simulink model "scara_controller_speed_control"  (R2013a)
settings: Solver=ode1  SolverMode=SingleTasking  StartTime=0.0  StopTime=inf  RelTol=1e-3
PreLoadFcn:
  | waijung.modelPreload; % Required for working with Waijung Blockset. Do not remove.
undefined symbols (not defined in the file or in its folder): ARM, disable_customio, enable_customio, fdesignblkfcn, gcbh, in1, in2, Link, LQFP100, MDK, out1, out2, out3, out4, out5, out6, output_customio, ST, STM32F407VG, STM32F4DISCOVERY
libraries: simulink x6, stm32f4_io_lib x3, USBVCP_STM32F4 x2, waijung_customcode x1, stm32f4_adc_lib x1, stm32f4_device_config_lib x1
CloseFcn:
  | waijung.modelClose; % Required for working with Waijung Blockset. Do not remove.
settings Model: Creator=Sr Antonio  LastModifiedBy=sp
settings DataIOCC: SignalLoggingSaveFormat=ModelDataLogs
settings OptimizationCC: ExpressionDepthLimit=2147483647  OptimizeModelRefInitCode=on  LifeSpan=1
settings DebuggingCC: MultiTaskDSMMsg=warning  FcnCallInpInsideContextMsg=EnableAllAsWarning
settings HardwareCC: ProdEndianess=LittleEndian  ProdHWDeviceType=ARM Compatible->Cortex - M4  TargetEndianess=LittleEndian  TargetHWDeviceType=ARM Compatible->Cortex - M4
settings RTWCC: SystemTargetFile=stm32f4.tlc  GenerateMakefile=off  TemplateMakefile=ert_default_tmf  Description=STM32F4 Target  ProcessScript=stm32f4_make_rtw_hook  RTWUseSimCustomCode=on
settings CodeAppCC: IgnoreCustomStorageClasses=off  CustomSymbolStrType=$N$R$M  InternalIdentifier=Classic
settings STFCustomTargetCC: ModelReferenceCompliant=off  CombineOutputUpdateFcns=on  ERTCustomFileBanners=on  SupportNonInlinedSFcns=off  MATLABClassNameForMDSCustomization=Simulink.SoftwareTarget.ERTCustomization  SystemTargetFile=stm32f4.tlc
settings ERTTargetCC: GenerateSampleERTMain=off  ModelReferenceCompliant=off  ParMdlRefBuildCompliant=off  CompOptLevelCompliant=off  ConcurrentExecutionCompliant=off  ERTFirstTimeCompliant=off  SupportContinuousTime=on  ModelStepFunctionPrototypeControlCompliant=off  CPPClassGenCompliant=off  ExtModeMexFile=noextcomm  ERTSrcFileBannerTemplate=stm32f4_code_template.cgt  ERTHdrFileBannerTemplate=stm32f4_code_template.cgt  ERTDataSrcFileTemplate=stm32f4_code_template.cgt  ERTDataHdrFileTemplate=stm32f4_code_template.cgt  ERTCustomFileTemplate=stm32f4_file_process.tlc

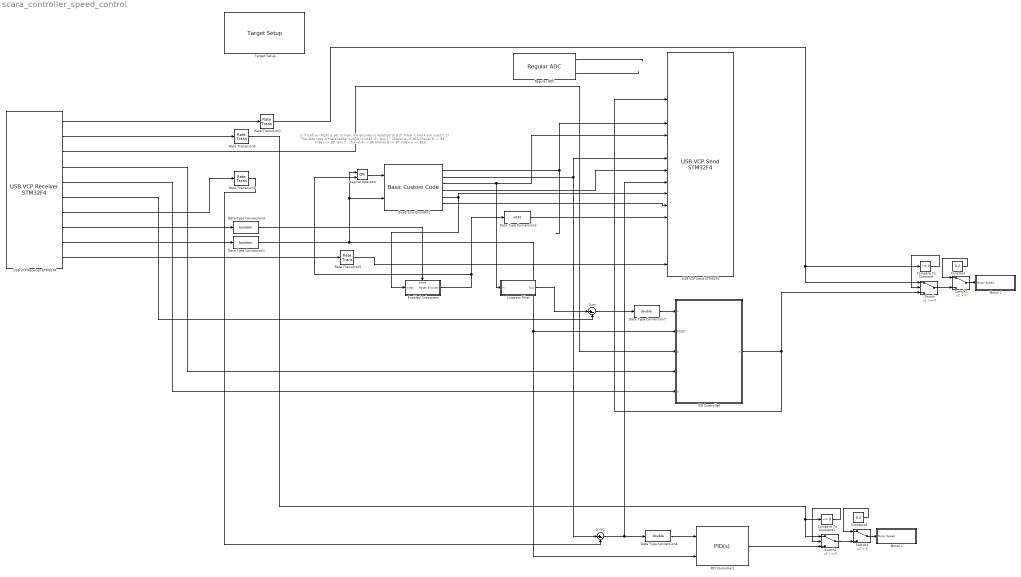
== system scara_controller_speed_control ==
  note: 1) if rLeft or rRight is set to high, the encoder is resetted to 0
      | 2) Timer 2 and 4 are used!!!
      | 2) The data type of the encoder output is int32.
      | 3) "enc 1": 	Chanel A --> A15
      | 		       Chanel B --> B3
      | 			Index --> D0
      |   "enc 2": 	Chanel A --> B6
      | 		       Chanel B --> B7
      | 			Index-> --> B12
  Compare To Constant : simulink/Logic and Bit Operations/Compare To Constant  relop=~=  const=0  OutDataTypeStr=boolean
  Compare To Constant1 : simulink/Logic and Bit Operations/Compare To Constant  relop=~=  const=0  OutDataTypeStr=boolean
  Constant : Constant  Value=0.2
  Constant2 : Constant  Value=0.2
  Data Type Conversion1 : DataTypeConversion  OutDataTypeStr=boolean
  Data Type Conversion2 : DataTypeConversion  OutDataTypeStr=int32
  Data Type Conversion3 : DataTypeConversion  OutDataTypeStr=boolean
  Data Type Conversion4 : DataTypeConversion  OutDataTypeStr=double
  Data Type Conversion7 : DataTypeConversion  OutDataTypeStr=double
  Enabled Subsystem : Subsystem  TreatAsAtomicUnit=on
  Logical Operator : Logic  Operator=OR  AllPortsSameDT=off  OutDataTypeStr=boolean
  Lowpass Filter : Subsystem  DialogController=fdesignblkfcn  InitFcn=fdesignblkfcn(gcbh, {'InitFcn'});  mask(Lowpass Filter){}
      mask help: Design a lowpass filter
      settings: CopyFcn=fdesignblkfcn(gcbh, {'CopyFcn'});
      mask Help: helpview(mapfilelocation('dsp'), 'dsplowpassfilter');
      mask Display: disp('Lowpass')
  Motor 1 : Subsystem
  Motor 2 : Subsystem
  PID Controller : Subsystem  DialogController=pidpack.PIDConfig.pidDDGCreate  mask(PID 1dof){Controller=PID, TimeDomain=Continuous-time, SampleTime=1, IntegratorMethod=Forward Euler, FilterMethod=Forward Euler, Form=Parallel, P=0.0005, I=0.0005, D=0, N=20, InitialConditionSource=internal, InitialConditionForIntegrator=0, InitialConditionForFilter=0, ExternalReset=rising, IgnoreLimit=off, ZeroCross=on, LimitOutput=on, UpperSaturationLimit=1, LowerSaturationLimit=-1, LinearizeAsGain=on, AntiWindupMode=clamping, Kb=1, TrackingMode=off, Kt=1, RndMeth=Floor, SaturateOnIntegerOverflow=off, LockScale=off, PParamMin=[], PParamMax=[], PParamDataTypeStr=Inherit: Inherit via internal rule, IParamMin=[], IParamMax=[], IParamDataTypeStr=Inherit: Inherit via internal rule, DParamMin=[], DParamMax=[], DParamDataTypeStr=Inherit: Inherit via internal rule, NParamMin=[], NParamMax=[], NParamDataTypeStr=Inherit: Inherit via internal rule, KbParamMin=[], KbParamMax=[], KbParamDataTypeStr=Inherit: Inherit via internal rule, KtParamMin=[], KtParamMax=[], KtParamDataTypeStr=Inherit: Inherit via internal rule, POutMin=[], POutMax=[], POutDataTypeStr=Inherit: Inherit via internal rule, IOutMin=[], IOutMax=[], IOutDataTypeStr=Inherit: Inherit via internal rule, DOutMin=[], DOutMax=[], DOutDataTypeStr=Inherit: Inherit via internal rule, NOutMin=[], NOutMax=[], NOutDataTypeStr=Inherit: Inherit via internal rule, KbOutMin=[], KbOutMax=[], KbOutDataTypeStr=Inherit: Inherit via internal rule, KtOutMin=[], KtOutMax=[], KtOutDataTypeStr=Inherit: Inherit via internal rule, IntegratorOutMin=[], IntegratorOutMax=[], IntegratorOutDataTypeStr=Inherit: Inherit via internal rule, FilterOutMin=[], FilterOutMax=[], FilterOutDataTypeStr=Inherit: Inherit via internal rule, SumOutMin=[], SumOutMax=[], SumOutDataTypeStr=Inherit: Inherit via internal rule, SumI1OutMin=[], SumI1OutMax=[], SumI1OutDataTypeStr=Inherit: Inherit via internal rule, SumI2OutMin=[], SumI2OutMax=[], SumI2OutDataTypeStr=Inherit: Inherit via internal rule, SumI3OutMin=[], SumI3OutMax=[], SumI3OutDataTypeStr=Inherit: Inherit via internal rule, SumDOutMin=[], SumDOutMax=[], SumDOutDataTypeStr=Inherit: Inherit via internal rule, SumAccumDataTypeStr=Inherit: Inherit via internal rule, SumI1AccumDataTypeStr=Inherit: Inherit via internal rule, SumI2AccumDataTypeStr=Inherit: Inherit via internal rule, SumI3AccumDataTypeStr=Inherit: Inherit via internal rule, SumDAccumDataTypeStr=Inherit: Inherit via internal rule, SaturationOutMin=[], SaturationOutMax=[], SaturationOutDataTypeStr=Inherit: Same as input, IntegratorContinuousStateAttributes='', IntegratorStateIdentifier=, IntegratorStateMustResolveToSignalObject=off, IntegratorRTWStateStorageClass=Auto, IntegratorRTWStateStorageTypeQualifier=, FilterContinuousStateAttributes='', FilterStateIdentifier=, FilterStateMustResolveToSignalObject=off, FilterRTWStateStorageClass=Auto, FilterRTWStateStorageTypeQualifier=}
      mask prompts: Controller "Simulink:masks:Controller_MP"; TimeDomain "Simulink:masks:TimeDomain_MP"; SampleTime "Simulink:masks:SampleTime1ForInherited_MP"; IntegratorMethod "Simulink:masks:IntegratorMethod_MP"; FilterMethod "Simulink:masks:FilterMethod_MP"; Form "Simulink:masks:Form_MP"; P "Simulink:masks:ProportionalP_MP"; I "Simulink:masks:IntegralI_MP"; D "Simulink:masks:DerivativeD_MP"; N "Simulink:masks:FilterCoefficientN_MP"; InitialConditionSource "Simulink:masks:Source_MP"; InitialConditionForIntegrator "Simulink:masks:Integrator_MP"; InitialConditionForFilter "Simulink:masks:Filter_MP"; ExternalReset "Simulink:masks:ExternalReset_MP"; IgnoreLimit "Simulink:masks:IgnoreResetWhenLinearizing_MP"; ZeroCross "Simulink:masks:EnableZerocrossingDetection_MP"; LimitOutput "Simulink:masks:LimitOutput_MP"; UpperSaturationLimit "Simulink:masks:UpperSaturationLimit_MP"; LowerSaturationLimit "Simulink:masks:LowerSaturationLimit_MP"; LinearizeAsGain "Simulink:masks:IgnoreSaturationWhenLinearizing_MP"; AntiWindupMode "Simulink:masks:AntiwindupMethod_MP"; Kb "Simulink:masks:BackcalculationCoefficientKb_MP"; TrackingMode "Simulink:masks:EnableTrackingMode_MP"; Kt "Simulink:masks:TrackingCoefficientKt_MP"; RndMeth "Simulink:masks:IntegerRoundingMode_MP"; SaturateOnIntegerOverflow "Simulink:masks:SaturateOnIntegerOverflow_MP"; LockScale "Simulink:masks:LockDataTypeAgainstFxpTools_MP"; PParamMin "Simulink:masks:PParameterMinimum_MP"; PParamMax "Simulink:masks:PParameterMaximum_MP"; PParamDataTypeStr "Simulink:masks:PParameter_MP"; IParamMin "Simulink:masks:IParameterMinimum_MP"; IParamMax "Simulink:masks:IParameterMaximum_MP"; IParamDataTypeStr "Simulink:masks:IParameter_MP"; DParamMin "Simulink:masks:DParameterMinimum_MP"; DParamMax "Simulink:masks:DParameterMaximum_MP"; DParamDataTypeStr "Simulink:masks:DParameter_MP"; NParamMin "Simulink:masks:NParameterMinimum_MP"; NParamMax "Simulink:masks:NParameterMaximum_MP"; NParamDataTypeStr "Simulink:masks:NParameter_MP"; KbParamMin "Simulink:masks:KbParameterMinimum_MP"; KbParamMax "Simulink:masks:KbParameterMaximum_MP"; KbParamDataTypeStr "Simulink:masks:KbParameter_MP"; KtParamMin "Simulink:masks:KtParameterMinimum_MP"; KtParamMax "Simulink:masks:KtParameterMaximum_MP"; KtParamDataTypeStr "Simulink:masks:KtParameter_MP"; POutMin "Simulink:masks:PProductOutputMinimum_MP"; POutMax "Simulink:masks:PProductOutputMaximum_MP"; POutDataTypeStr "Simulink:masks:PProductOutput_MP"; IOutMin "Simulink:masks:IProductOutputMinimum_MP"; IOutMax "Simulink:masks:IProductOutputMaximum_MP"; IOutDataTypeStr "Simulink:masks:IProductOutput_MP"; DOutMin "Simulink:masks:DProductOutputMinimum_MP"; DOutMax "Simulink:masks:DProductOutputMaximum_MP"; DOutDataTypeStr "Simulink:masks:DProductOutput_MP"; NOutMin "Simulink:masks:NProductOutputMinimum_MP"; NOutMax "Simulink:masks:NProductOutputMaximum_MP"; NOutDataTypeStr "Simulink:masks:NProductOutput_MP"; KbOutMin "Simulink:masks:KbProductOutputMinimum_MP"; KbOutMax "Simulink:masks:KbProductOutputMaximum_MP"; KbOutDataTypeStr "Simulink:masks:KbProductOutput_MP"; KtOutMin "Simulink:masks:KtProductOutputMinimum_MP"; KtOutMax "Simulink:masks:KtProductOutputMaximum_MP"; KtOutDataTypeStr "Simulink:masks:KtProductOutput_MP"; IntegratorOutMin "Simulink:masks:IntegratorOutputMinimum_MP"; IntegratorOutMax "Simulink:masks:IntegratorOutputMaximum_MP"; IntegratorOutDataTypeStr "Simulink:masks:IntegratorOutput_MP"; FilterOutMin "Simulink:masks:FilterOutputMinimum_MP"; FilterOutMax "Simulink:masks:FilterOutputMaximum_MP"; FilterOutDataTypeStr "Simulink:masks:FilterOutput_MP"; SumOutMin "Simulink:masks:SumOutputMinimum_MP"; SumOutMax "Simulink:masks:SumOutputMaximum_MP"; SumOutDataTypeStr "Simulink:masks:SumOutput_MP"; SumI1OutMin "Simulink:masks:SumI1OutputMinimum_MP"; SumI1OutMax "Simulink:masks:SumI1OutputMaximum_MP"; SumI1OutDataTypeStr "Simulink:masks:SumI1Output_MP"; SumI2OutMin "Simulink:masks:SumI2OutputMinimum_MP"; SumI2OutMax "Simulink:masks:SumI2OutputMaximum_MP"; SumI2OutDataTypeStr "Simulink:masks:SumI2Output_MP"; SumI3OutMin "Simulink:masks:SumI3OutputMinimum_MP"; SumI3OutMax "Simulink:masks:SumI3OutputMaximum_MP"; SumI3OutDataTypeStr "Simulink:masks:SumI3Output_MP"; SumDOutMin "Simulink:masks:SumDOutputMinimum_MP"; SumDOutMax "Simulink:masks:SumDOutputMaximum_MP"; SumDOutDataTypeStr "Simulink:masks:SumDOutput_MP"; SumAccumDataTypeStr "Simulink:masks:AccumulatorOfSum_MP"; SumI1AccumDataTypeStr "Simulink:masks:AccumulatorOfSumI1_MP"; SumI2AccumDataTypeStr "Simulink:masks:AccumulatorOfSumI2_MP"; SumI3AccumDataTypeStr "Simulink:masks:AccumulatorOfSumI3_MP"; SumDAccumDataTypeStr "Simulink:masks:AccumulatorOfSumD_MP"; SaturationOutMin "Simulink:masks:SaturationOutputMinimum_MP"; SaturationOutMax "Simulink:masks:SaturationOutputMaximum_MP"; SaturationOutDataTypeStr "Simulink:masks:SaturationOutput_MP"; IntegratorContinuousStateAttributes "Simulink:masks:StateNameegposition_MP"; IntegratorStateIdentifier "Simulink:masks:StateName_MP"; IntegratorStateMustResolveToSignalObject "Simulink:masks:StateNameMustResolveToSimulinkSignalObject_MP"; IntegratorRTWStateStorageClass "Simulink:masks:CodeGenerationStorageClass_MP"; IntegratorRTWStateStorageTypeQualifier "Simulink:masks:CodeGenerationStorageTypeQualifier_MP"; FilterContinuousStateAttributes "Simulink:masks:StateNameegposition_MP"; FilterStateIdentifier "Simulink:masks:StateName_MP"; FilterStateMustResolveToSignalObject "Simulink:masks:StateNameMustResolveToSimulinkSignalObject_MP"; FilterRTWStateStorageClass "Simulink:masks:CodeGenerationStorageClass_MP"; FilterRTWStateStorageTypeQualifier "Simulink:masks:CodeGenerationStorageTypeQualifier_MP"
      mask help: Simulink:masks:PID1dof_MD
      mask init:
      | pidpack.PIDConfig.configPID(gcbh);
      settings: DeleteFcn=pidpack.PIDConfig.closeTuner(gcbh)  ModelCloseFcn=pidpack.PIDConfig.closeTuner(gcbh)  NameChangeFcn=pidpack.PIDConfig.updateTunerName(gcbh)
      mask TypeOptions Controller: Simulink:masks:PID | Simulink:masks:PI | Simulink:masks:PD | Simulink:masks:P | Simulink:masks:I
      mask TypeOptions TimeDomain: Simulink:masks:ContinuousTime | Simulink:masks:DiscreteTime
      mask TypeOptions IntegratorMethod: Simulink:masks:ForwardEuler | Simulink:masks:BackwardEuler | Simulink:masks:Trapezoidal
      mask TypeOptions FilterMethod: Simulink:masks:ForwardEuler | Simulink:masks:BackwardEuler | Simulink:masks:Trapezoidal
      mask TypeOptions Form: Simulink:masks:Ideal | Simulink:masks:Parallel
      mask TypeOptions InitialConditionSource: Simulink:masks:internal | Simulink:masks:external
      mask TypeOptions ExternalReset: Simulink:masks:none | Simulink:masks:rising | Simulink:masks:falling | Simulink:masks:either | Simulink:masks:level
      mask TypeOptions AntiWindupMode: Simulink:masks:none | Simulink:masks:backCalculation | Simulink:masks:clamping
      mask TypeOptions RndMeth: Simulink:masks:Ceiling | Simulink:masks:Convergent | Simulink:masks:Floor | Simulink:masks:Nearest | Simulink:masks:Round | Simulink:masks:Simplest | Simulink:masks:Zero
      mask TypeOptions IntegratorRTWStateStorageClass: Simulink:masks:Auto | Simulink:masks:ExportedGlobal | Simulink:masks:ImportedExtern | Simulink:masks:ImportedExternPointer
      mask TypeOptions FilterRTWStateStorageClass: Simulink:masks:Auto | Simulink:masks:ExportedGlobal | Simulink:masks:ImportedExtern | Simulink:masks:ImportedExternPointer
      mask Display:
      | image(imread(fullfile(matlabroot,'toolbox','simulink','blocks','@pidpack','@PIDMasks','images','blank.png'),'png'),[0 0 1 1]);
      | disp('PID(s)')
      | port_label('input',1, '');
      | port_label('output',1, '');
      | plot([0 4 4 7]+2,[0 0 8 8]+208);
      | plot([1 4 6]+2,[3 6 3]+208);
      | plot([0 4 6 10]+182,[0 0 8 8]+148);
  PID Controller1 : simulink/Continuous/PID Controller  Controller=PID  TimeDomain=Continuous-time  SampleTime=1  IntegratorMethod=Forward Euler  FilterMethod=Forward Euler  Form=Parallel  P=0.0005  I=0.0005  D=0  N=100  InitialConditionSource=internal  InitialConditionForIntegrator=0  InitialConditionForFilter=0  ExternalReset=rising  LimitOutput=on  UpperSaturationLimit=1  LowerSaturationLimit=-1  LinearizeAsGain=on  AntiWindupMode=clamping  Kb=1  TrackingMode=off  Kt=1  PParamMin=[]  PParamMax=[]  IParamMin=[]  IParamMax=[]  DParamMin=[]  DParamMax=[]  NParamMin=[]  NParamMax=[]  KbParamMin=[]  KbParamMax=[]  KtParamMin=[]  KtParamMax=[]  POutMin=[]  POutMax=[]  IOutMin=[]  IOutMax=[]  DOutMin=[]  DOutMax=[]  NOutMin=[]  NOutMax=[]  KbOutMin=[]  KbOutMax=[]  KtOutMin=[]  KtOutMax=[]  IntegratorOutMin=[]  IntegratorOutMax=[]  FilterOutMin=[]  FilterOutMax=[]  SumOutMin=[]  SumOutMax=[]  SumI1OutMin=[]  SumI1OutMax=[]  SumI2OutMin=[]  SumI2OutMax=[]  SumI3OutMin=[]  SumI3OutMax=[]  SumDOutMin=[]  SumDOutMax=[]  SaturationOutMin=[]  SaturationOutMax=[]  IntegratorContinuousStateAttributes=''  IntegratorStateMustResolveToSignalObject=off  IntegratorRTWStateStorageClass=Auto  FilterContinuousStateAttributes=''  FilterStateMustResolveToSignalObject=off  FilterRTWStateStorageClass=Auto
  Quadratur Encoder2 : waijung_customcode/Basic Custom Code  inputporttype=boolean,boolean  cinputportlabel=resetEncoder1, resetEncoder2  cinputportlabelstr="[\"resetEncoder1\",\" resetEncoder2\"]"  inputportcount=2  inputporttypeid="[8  8]"  outputporttype=int32,int32,int32,int32,int32,int32  coutputportlabel=encoder1, encoder2, encoder1_speed, encoder2_speed, encoder1_index, encoder2_index  coutputportlabelstr="[\"encoder1\",\" encoder2\",\" encoder1_speed\",\" encoder2_speed\",\" encoder1_index\",\" encoder2_index\"]"  outputportcount=6  outputporttypeid="[6  6  6  6  6  6]"  incpath={fullfile(pwd,'customcode')}  srcpath={fullfile(pwd,'customcode')}  incfiles={''}  srcfiles={'stm32f4_io_customcode.c'}  enablefuncallstr=enable_customio();  outputfuncallstr=output_customio(in1,in2,out1,out2,out3,out4,out5,out6);  disablefuncallstr=disable_customio();  sampletime=0.001  sampletimestr=0.001  blockid=QuadraturEncoder2  enablecustomportlabel=on  incfilestrarray="[\"\"]"  inputportdiminfo="[1  1  1  8;1  1  1  8]"  outputportdiminfo="[1  1  1  6;1  1  1  6;1  1  1  6;1  1  1  6;1  1  1  6;1  1  1  6]"
  Rate Transition1 : RateTransition  Integrity=off  Deterministic=off  OutPortSampleTime=0.001
  Rate Transition3 : RateTransition  OutPortSampleTime=0.01
  Rate Transition4 : RateTransition  Integrity=off  Deterministic=off  OutPortSampleTime=0.001
  Rate Transition5 : RateTransition  OutPortSampleTime=0.01
  Regular ADC : stm32f4_adc_lib/Regular ADC  adcmodule=1  outputdatatype=Double  prescaler=2  prescalerstr=ADC_Prescaler_Div2  chsamplingtime=Auto  chsamplingtimestr=ADC_SampleTime_480Cycles  read_an0=off  read_an1=off  read_an2=off  read_an3=off  read_an4=off  read_an5=on  read_an6=off  read_an7=off  read_an8=off  read_an9=off  read_an10=off  read_an11=off  read_an12=off  read_an13=off  read_an14=off  read_an15=off  read_an16=off  read_an17=on  read_an18=off  pinstr=GPIO_Pin_5  usedpinarray="[0  0  0  0  0  1  0  0  0  0  0  0  0  0  0  0  0  1  0]"  usedportidarray=[0]  usedpinidarray=[5]  usedpinidcount=1  sampletime=0.01  blockid=RegularADC  enablecustomportlabel=on  cinputportlabel=0  coutputportlabel=Motor1Current, BoardTemp
  Sum : Sum  Inputs=|+-  AccumDataTypeStr=int32
  Sum1 : Sum  Inputs=|+-  AccumDataTypeStr=int32
  Switch : Switch
  Switch1 : Switch
  Switch2 : Switch  Criteria=u2 > Threshold
  Switch4 : Switch  Criteria=u2 > Threshold
  Target Setup : stm32f4_device_config_lib/Target Setup  Priority=100  compiler=MDK-ARM  previous_compiler=MDK-ARM  mcu=STM32F407VG (LQFP100); STM32F4DISCOVERY  mcustr=STM32F407VG  clockconfig=STM32F4DISCOVERY Default (HSEOSC-8MHz/HCLK-168MHz)  system_stm32f4xx_c_path=C:\Program Files\MATLAB\waijung14_12a\targets\stm32f4_target\stm32f4\utils\STM32F4xx_AN3988_V1.0.1\stm32f4_default\hseosc8mhz  showmemoryconfiguration=on  stacksize=0x2000  heapsize=0x2000  enableautocompiledownload=on  fullchiperase=off  programmerinterface=ST-Link  editctrlstr=on  compilercontrolstr=-c --cpu Cortex-M4.fp -g -O3 --apcs=interwork --split_sections $(INCLUDES)  assemblercontrolstr="--cpu Cortex-M4.fp -g --apcs=interwork  --xref $(INCLUDES)"  linkercontrolstr="--cpu Cortex-M4.fp --strict --scatter \"$(MODELNAME).sct\" --summary_stderr --info summarysizes --map --xref --callgraph --symbols --info sizes --info totals --info unused --info veneers  --list \".\\$(MODELNAME).map\" -o $(MODELNAME).axf"  runafterdownload=on  execprofile=None  profileruart=1  profilerbaud=115200  profilertxpin=Not used  profilerinitstr=0.001,168000000,168000,115200,0  manualsetsampletime=off  sampletime=0.001  blockid=TargetSetup  systickreloadvalue=168000  hseval=8000000  lastprofileruart=1  hclk=168000000  flashorigin=0x08000000  flashlength=0x00100000  ramorigin=0x20000000  ramlength=0x00020000  useextram=off
  USB VCP Receiver STM32F4 : USBVCP_STM32F4/USB VCP Receiver STM32F4  speed="USB 1.1   12Mbit/s"  data_size=2048 Bytes  header_data='7E 7E'  binary_data='double double double double double int32 int32 int32 int32 int32'  terminator_data='03 03'  sampletime=0.001
  USB VCP Send STM32F1 : USBVCP_STM32F4/USB VCP Send STM32F4  speed="USB 1.1   12Mbit/s"  data_size=2048 Bytes  header_data='0E 0E'  binary_data='double double double double int32 int32 int32 int32 int32 int32 int32 int32 int32 int32 int32 int32 int32 int32'  terminator_data='0A 0A'  sampletime=0.001
  wires:
  USB VCP Receiver STM32F4/1 -> Rate Transition1/1
  Quadratur Encoder2/1 -> USB VCP Send STM32F1/6
  PID Controller/1(y) -> Switch/3, USB VCP Send STM32F1/4
  Sum/1 -> Data Type Conversion7/1
  Switch/1 -> Switch2/3
  Compare To Constant/1 -> Switch/2
  Quadratur Encoder2/2 -> USB VCP Send STM32F1/9, Sum1/1
  PID Controller1/1 -> Switch1/3
  Rate Transition3/1 -> Sum1/2
  Sum1/1 -> Data Type Conversion4/1, USB VCP Send STM32F1/11
  Data Type Conversion4/1 -> PID Controller1/1
  Data Type Conversion1/1 -> Quadratur Encoder2/2, Logical Operator/1, PID Controller1/2, PID Controller/2(RESET)
  Switch1/1 -> Switch4/3
  Compare To Constant1/1 -> Switch1/2
  USB VCP Receiver STM32F4/7 -> Rate Transition3/1
  USB VCP Receiver STM32F4/2 -> Rate Transition4/1
  USB VCP Receiver STM32F4/9 -> Data Type Conversion1/1
  Quadratur Encoder2/3 -> USB VCP Send STM32F1/7, Lowpass Filter/1(In)
  Quadratur Encoder2/4 -> USB VCP Send STM32F1/10
  Rate Transition1/1 -> Switch/1, Compare To Constant/1
  Rate Transition4/1 -> Switch1/1, Compare To Constant1/1
  Data Type Conversion7/1 -> PID Controller/1(u)
  Quadratur Encoder2/5 -> USB VCP Send STM32F1/12, Enabled Subsystem/1(Index)
  Quadratur Encoder2/6 -> USB VCP Send STM32F1/13
  Enabled Subsystem/1(Reset Encoder) -> Data Type Conversion2/1, Logical Operator/2
  Logical Operator/1 -> Quadratur Encoder2/1
  USB VCP Receiver STM32F4/8 -> Data Type Conversion3/1
  Constant/1 -> Switch2/1
  Switch2/1 -> Motor 2/1(Motor Speed)
  Data Type Conversion2/1 -> USB VCP Send STM32F1/14
  USB VCP Receiver STM32F4/6 -> Sum/2
  USB VCP Receiver STM32F4/10 -> Rate Transition5/1
  Rate Transition5/1 -> USB VCP Send STM32F1/18
  Constant2/1 -> Switch4/1
  Switch4/1 -> Motor 1/1(Motor Speed)
  Data Type Conversion3/1 -> Enabled Subsystem/Enable
  USB VCP Receiver STM32F4/3 -> PID Controller/3(p)
  USB VCP Receiver STM32F4/4 -> PID Controller/4(i)
  USB VCP Receiver STM32F4/5 -> PID Controller/5(d)
  Regular ADC/1 -> ?
  Regular ADC/2 -> ?
  Lowpass Filter/1(Out) -> Sum/1
  ? -> USB VCP Send STM32F1/8

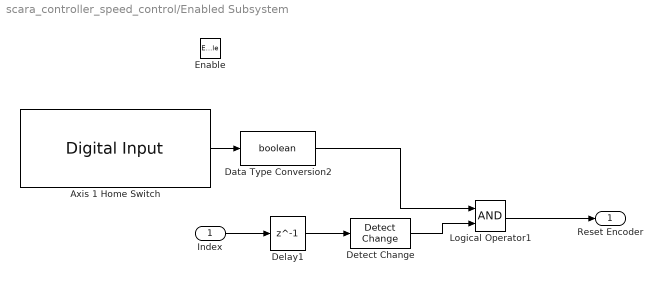
== system scara_controller_speed_control/Enabled Subsystem ==
  Index : Inport
  Enable : EnablePort
  Axis 1 Home Switch : stm32f4_io_lib/Digital Input  port=A  speed=100  porttype=None  porttypestr=NOPULL  use_pin0=off  use_pin1=off  use_pin2=off  use_pin3=off  use_pin4=off  use_pin5=off  use_pin6=off  use_pin7=off  use_pin8=off  use_pin9=off  use_pin10=on  use_pin11=off  use_pin12=off  use_pin13=off  use_pin14=off  use_pin15=off  pinstr=GPIO_Pin_10  usedpinarray="[0  0  0  0  0  0  0  0  0  0  1  0  0  0  0  0]"  bitbandingstr="#define EnabledSubsystemAxis1HomeSwitch_A10 Peripheral_BB(GPIOA->IDR, 10)  /* Output pin */"  sampletime=0.01  sampletimestr=0.01  blockid=EnabledSubsystemAxis1HomeSwitch  enablecustomportlabel=off  glabalinit=off  cinputportlabel=In1, In2  coutputportlabel=Out1, Out2
  Data Type Conversion2 : DataTypeConversion  OutDataTypeStr=boolean
  Delay1 : Delay  DelayLength=1  InitialCondition=0
  Detect Change : simulink/Logic and Bit Operations/Detect Change  vinit=0  InputProcessing=Inherited  OutDataTypeStr=boolean
  Logical Operator1 : Logic  AllPortsSameDT=off  OutDataTypeStr=boolean
  Reset Encoder : Outport  OutputWhenDisabled=reset  InitialOutput=[0]
  wires:
  Detect Change/1 -> Logical Operator1/2
  Delay1/1 -> Detect Change/1
  Index/1 -> Delay1/1
  Logical Operator1/1 -> Reset Encoder/1
  Axis 1 Home Switch/1 -> Data Type Conversion2/1
  Data Type Conversion2/1 -> Logical Operator1/1

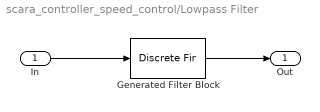
== system scara_controller_speed_control/Lowpass Filter ==
  In : Inport
  Generated Filter Block : DiscreteFir  Tag=BlockMethodSubSystem  Coefficients=[-0.0024228738523269142 -0.002083244982079274 0.0067703446401187091 0.016731945423489058 0.011117076081077608 -0.0062311454141445394 -0.008401617186026911 0.0092567976151380175 0.012982883808855752 -0.010121234703278968 -0.018273518733782485 0.011431962071777957 0.02617588858040763 -0.012489027835322923 -0.037996623145463579 0.013388945199366963 0.058155465814729891 -0.014048043515808939 -0.10272466857882172 0.014462275771238358 0.31716649721769491 0.48538764678732504 0.31716649721769491 0.014462275771238358 -0.10272466857882172 -0.014048043515808939 0.058155465814729891 0.013388945199366963 -0.037996623145463579 -0.012489027835322923 0.02617588858040763 0.011431962071777957 -0.018273518733782485 -0.010121234703278968 0.012982883808855752 0.0092567976151380175 -0.008401617186026911 -0.0062311454141445394 0.011117076081077608 0.016731945423489058 0.0067703446401187091 -0.002083244982079274 -0.0024228738523269142]  InputProcessing=Columns as channels (frame based)
  Out : Outport
  wires:
  In/1 -> Generated Filter Block/1
  Generated Filter Block/1 -> Out/1

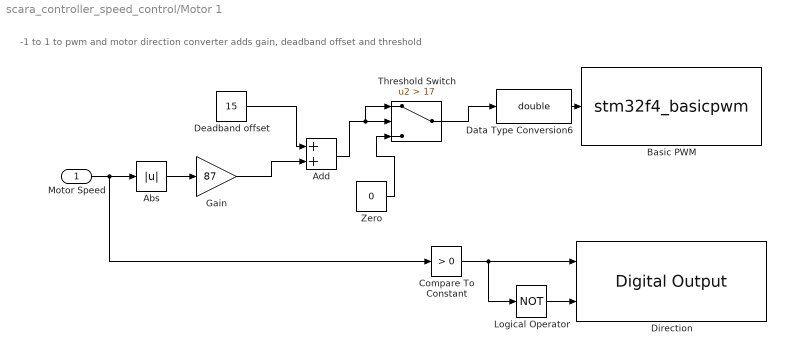
== system scara_controller_speed_control/Motor 1 ==
  note: -1 to 1 to pwm and motor direction converter
      | adds gain, deadband offset and threshold
  Motor Speed : Inport  OutMin=[-1]  OutMax=[1]  OutDataTypeStr=double
  Abs : Abs
  Add : Sum
  Basic PWM : S-Function  FunctionName=stm32f4_basicpwm  Parameters=timer,pwmperiod,ch1pin,ch2pin,ch3pin,ch4pin,sampletime,sampletimestr,blockid,apb,portstr,pinstr,pinmat,timarr,timprescale,chmat,polaritystr  EnableBusSupport=off  mask(stm32f4_basicpwm){timer=3, pwmperiod=4e-5, polarity=Active High, polaritystr=TIM_OCPolarity_High, ch1pin=A6, ch2pin=Not available - Do not use, ch3pin=Not available - Do not use, ch4pin=Not available - Do not use, sampletime=0.01, sampletimestr=0.01, blockid=Motor1BasicPWM, portpinstr=A6,,,, enablecustomportlabel=off, cinputportlabel=In1, In2, In3, In4, coutputportlabel=0, apb=1, portstr=["A"], pinstr=["GPIO_Pin_6"], pinmat=[1 6], timarr=1119, timprescale=2, chmat=[1]}
      mask prompts: pwmperiod "PWM Period (seconds)"; ch1pin "Channel 1"; ch2pin "Channel 2"; ch3pin "Channel 3"; ch4pin "Channel 4"; sampletime "Sample time (sec)"; sampletimestr "Compiled sample time (sec) in string"; portpinstr "Port pin string"; enablecustomportlabel "Enable custom port labels"; cinputportlabel "Custom input port labels (Ex. In1, In2, In3)"; coutputportlabel "Custom output port labels (Ex. Out1, Out2, Out3)"; portstr "Port string"; pinstr "Pin string"; pinmat "Pin matrix"; timarr "Timer ARR"; timprescale "Timer PRESCALE"; chmat "Channel order"
      mask help:
      | This block implements basic Edge-aligned Pulse Width Modulation (PWM) generation.
      | All timers are 16-bit. The PWM period is fixed (per timer).
      mask init:
      | stm32f4_basicpwm_callback('init');
      mask Help: web(fullfile(waijungdocroot,'stm32f4_basicpwm.htm'),'-browser')
      mask TypeOptions timer: 1 | 2 | 3 | 4 | 5 | 8 | 9 | 10 | 11 | 12 | 13 | 14
      mask Callback timer: stm32f4_basicpwm_callback('timer');
      mask Callback pwmperiod: stm32f4_basicpwm_callback('pwmperiod');
      mask TypeOptions polarity: Active High | Active Low
      mask Callback polarity: stm32f4_basicpwm_callback('polarity');
      mask TypeOptions ch1pin: Not available - Do not use | A6 | C6 | B4
      mask Callback ch1pin: stm32f4_basicpwm_callback('ch1pin');
      mask TypeOptions ch2pin: Not available - Do not use | A7 | C7 | B5
      mask Callback ch2pin: stm32f4_basicpwm_callback('ch2pin');
      mask TypeOptions ch3pin: Not available - Do not use | B0 | C8
      mask Callback ch3pin: stm32f4_basicpwm_callback('ch3pin');
      mask TypeOptions ch4pin: Not available - Do not use | B1 | C9
      mask Callback ch4pin: stm32f4_basicpwm_callback('ch4pin');
      mask Callback sampletime: stm32f4_basicpwm_callback('sampletime');
      mask Callback sampletimestr: stm32f4_basicpwm_callback('sampletimestr');
      mask Callback blockid: stm32f4_basicpwm_callback('blockid');
      mask Callback enablecustomportlabel: stm32f4_basicpwm_callback('enablecustomportlabel');
      mask Display: text(0.95, 0.5, 'Timer: 3\nPolarity: Active High\nPeriod (sec) 4e-5\nTs (sec): 0.01','ver','middle','hor','right');port_label('input', 1,'CH1 (A6)')
  Compare To Constant : simulink/Logic and Bit Operations/Compare To Constant  relop=>  const=0  OutDataTypeStr=boolean
  Data Type Conversion6 : DataTypeConversion  OutDataTypeStr=double
  Deadband offset : Constant  Value=15
  Direction : stm32f4_io_lib/Digital Output  use_bitband=on  port=A  speed=100  porttype=Push Pull  porttypestr=PP  use_pin0=off  use_pin1=off  use_pin2=off  use_pin3=off  use_pin4=on  use_pin5=on  use_pin6=off  use_pin7=off  use_pin8=off  use_pin9=off  use_pin10=off  use_pin11=off  use_pin12=off  use_pin13=off  use_pin14=off  use_pin15=off  pinstr=GPIO_Pin_4 | GPIO_Pin_5  usedpinarray="[0  0  0  0  1  1  0  0  0  0  0  0  0  0  0  0]"  bitbandingstr=|  sampletime=-1  sampletimestr=0  blockid=Motor1Direction  enablecustomportlabel=off  globalinit=off  cinputportlabel=In1, In2  coutputportlabel=0
      | #define Motor1Direction_A4 Peripheral_BB(GPIOA->ODR, 4)  /* Output pin */
      | #define Motor1Direction_A5 Peripheral_BB(GPIOA->ODR, 5)  /* Output pin */
  Gain : Gain  Gain=87
  Logical Operator : Logic  Operator=NOT  AllPortsSameDT=off  OutDataTypeStr=boolean
  Threshold Switch : Switch  Criteria=u2 > Threshold  Threshold=17
  Zero : Constant  Value=0
  wires:
  Logical Operator/1 -> Direction/2
  Add/1 -> Threshold Switch/1, Threshold Switch/2
  Compare To Constant/1 -> Direction/1, Logical Operator/1
  Motor Speed/1 -> Abs/1, Compare To Constant/1
  Deadband offset/1 -> Add/1
  Gain/1 -> Add/2
  Data Type Conversion6/1 -> Basic PWM/1
  Abs/1 -> Gain/1
  Threshold Switch/1 -> Data Type Conversion6/1
  Zero/1 -> Threshold Switch/3

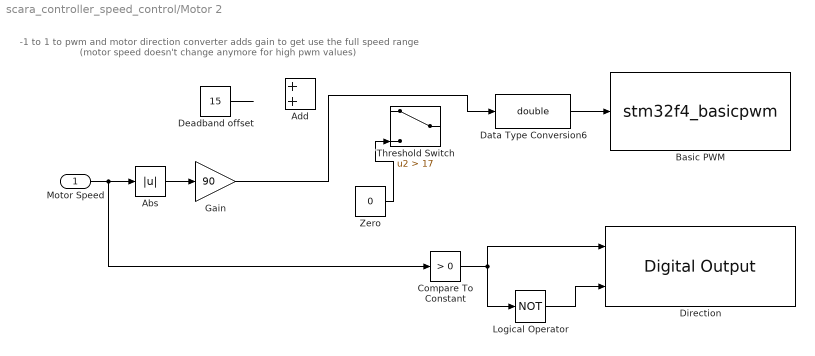
== system scara_controller_speed_control/Motor 2 ==
  note: -1 to 1 to pwm and motor direction converter
      | adds gain to get use the full speed range (motor speed doesn't change anymore for high pwm values)
  Motor Speed : Inport  OutMin=[-1]  OutMax=[1]  OutDataTypeStr=double
  Abs : Abs
  Add : Sum
  Basic PWM : S-Function  FunctionName=stm32f4_basicpwm  Parameters=timer,pwmperiod,ch1pin,ch2pin,ch3pin,ch4pin,sampletime,sampletimestr,blockid,apb,portstr,pinstr,pinmat,timarr,timprescale,chmat,polaritystr  EnableBusSupport=off  mask(stm32f4_basicpwm){timer=5, pwmperiod=4e-5, polarity=Active High, polaritystr=TIM_OCPolarity_High, ch1pin=A0, ch2pin=Not available - Do not use, ch3pin=Not available - Do not use, ch4pin=Not available - Do not use, sampletime=0.01, sampletimestr=0.01, blockid=Motor2BasicPWM, portpinstr=A0,,,, enablecustomportlabel=off, cinputportlabel=In1, In2, In3, In4, coutputportlabel=0, apb=1, portstr=["A"], pinstr=["GPIO_Pin_0"], pinmat=[1 0], timarr=1119, timprescale=2, chmat=[1]}
      mask prompts: pwmperiod "PWM Period (seconds)"; ch1pin "Channel 1"; ch2pin "Channel 2"; ch3pin "Channel 3"; ch4pin "Channel 4"; sampletime "Sample time (sec)"; sampletimestr "Compiled sample time (sec) in string"; portpinstr "Port pin string"; enablecustomportlabel "Enable custom port labels"; cinputportlabel "Custom input port labels (Ex. In1, In2, In3)"; coutputportlabel "Custom output port labels (Ex. Out1, Out2, Out3)"; portstr "Port string"; pinstr "Pin string"; pinmat "Pin matrix"; timarr "Timer ARR"; timprescale "Timer PRESCALE"; chmat "Channel order"
      mask help:
      | This block implements basic Edge-aligned Pulse Width Modulation (PWM) generation.
      | All timers are 16-bit. The PWM period is fixed (per timer).
      mask init:
      | stm32f4_basicpwm_callback('init');
      mask Help: web(fullfile(waijungdocroot,'stm32f4_basicpwm.htm'),'-browser')
      mask TypeOptions timer: 1 | 2 | 3 | 4 | 5 | 8 | 9 | 10 | 11 | 12 | 13 | 14
      mask Callback timer: stm32f4_basicpwm_callback('timer');
      mask Callback pwmperiod: stm32f4_basicpwm_callback('pwmperiod');
      mask TypeOptions polarity: Active High | Active Low
      mask Callback polarity: stm32f4_basicpwm_callback('polarity');
      mask TypeOptions ch1pin: Not available - Do not use | A0
      mask Callback ch1pin: stm32f4_basicpwm_callback('ch1pin');
      mask TypeOptions ch2pin: Not available - Do not use | A1
      mask Callback ch2pin: stm32f4_basicpwm_callback('ch2pin');
      mask TypeOptions ch3pin: Not available - Do not use | A2
      mask Callback ch3pin: stm32f4_basicpwm_callback('ch3pin');
      mask TypeOptions ch4pin: Not available - Do not use | A3
      mask Callback ch4pin: stm32f4_basicpwm_callback('ch4pin');
      mask Callback sampletime: stm32f4_basicpwm_callback('sampletime');
      mask Callback sampletimestr: stm32f4_basicpwm_callback('sampletimestr');
      mask Callback blockid: stm32f4_basicpwm_callback('blockid');
      mask Callback enablecustomportlabel: stm32f4_basicpwm_callback('enablecustomportlabel');
      mask Display: text(0.95, 0.5, 'Timer: 5\nPolarity: Active High\nPeriod (sec) 4e-5\nTs (sec): 0.01','ver','middle','hor','right');port_label('input', 1,'CH1 (A0)')
  Compare To Constant : simulink/Logic and Bit Operations/Compare To Constant  relop=>  const=0  OutDataTypeStr=boolean
  Data Type Conversion6 : DataTypeConversion  OutDataTypeStr=double
  Deadband offset : Constant  Value=15
  Direction : stm32f4_io_lib/Digital Output  use_bitband=on  port=A  speed=100  porttype=Push Pull  porttypestr=PP  use_pin0=off  use_pin1=on  use_pin2=off  use_pin3=on  use_pin4=off  use_pin5=off  use_pin6=off  use_pin7=off  use_pin8=off  use_pin9=off  use_pin10=off  use_pin11=off  use_pin12=off  use_pin13=off  use_pin14=off  use_pin15=off  pinstr=GPIO_Pin_1 | GPIO_Pin_3  usedpinarray="[0  1  0  1  0  0  0  0  0  0  0  0  0  0  0  0]"  bitbandingstr=|  sampletime=-1  sampletimestr=0  blockid=Motor2Direction  enablecustomportlabel=off  globalinit=off  cinputportlabel=In1, In2  coutputportlabel=0
      | #define Motor2Direction_A1 Peripheral_BB(GPIOA->ODR, 1)  /* Output pin */
      | #define Motor2Direction_A3 Peripheral_BB(GPIOA->ODR, 3)  /* Output pin */
  Gain : Gain  Gain=90
  Logical Operator : Logic  Operator=NOT  AllPortsSameDT=off  OutDataTypeStr=boolean
  Threshold Switch : Switch  Criteria=u2 > Threshold  Threshold=17
  Zero : Constant  Value=0
  wires:
  Logical Operator/1 -> Direction/2
  ? -> Threshold Switch/1, Threshold Switch/2
  Compare To Constant/1 -> Direction/1, Logical Operator/1
  Motor Speed/1 -> Abs/1, Compare To Constant/1
  Deadband offset/1 -> ?
  Abs/1 -> Gain/1
  Gain/1 -> Data Type Conversion6/1
  Zero/1 -> Threshold Switch/3
  Data Type Conversion6/1 -> Basic PWM/1

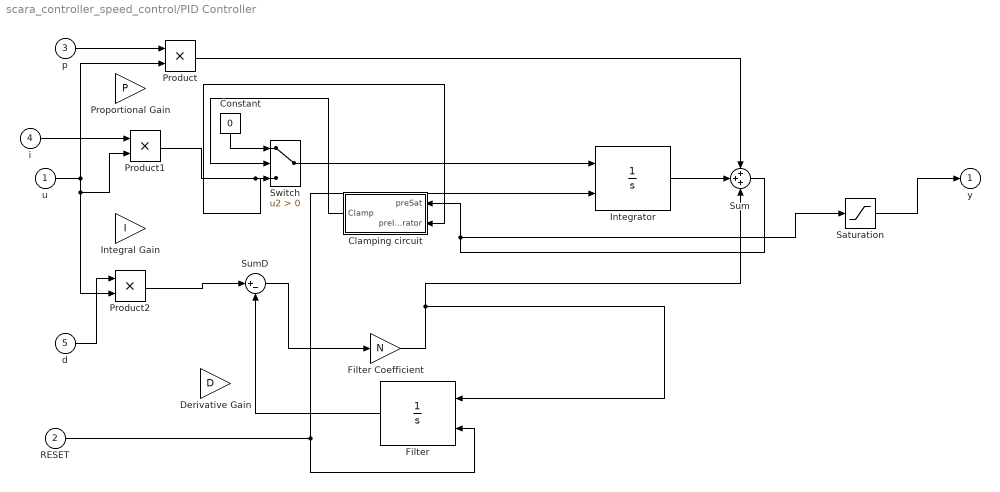
== system scara_controller_speed_control/PID Controller ==
  u : Inport
  RESET : Inport  Port=2
  p : Inport  Port=3
  i : Inport  Port=4
  d : Inport  Port=5
  Clamping circuit : Subsystem
  Constant : Constant  DisableCoverage=on  Value=0  OutDataTypeStr=Inherit: Inherit via back propagation  PreserveConstantTs=on
  Derivative Gain : Gain  DisableCoverage=on  Gain=D  ParamMin=DParamMin  ParamMax=DParamMax  ParamDataTypeStr=DParamDataTypeStr  OutMin=DOutMin  OutMax=DOutMax  OutDataTypeStr=DOutDataTypeStr
  Filter : Integrator  DisableCoverage=on  ExternalReset=rising  InitialCondition=InitialConditionForFilter
  Filter Coefficient : Gain  Gain=N  ParamMin=NParamMin  ParamMax=NParamMax  ParamDataTypeStr=NParamDataTypeStr  OutMin=NOutMin  OutMax=NOutMax  OutDataTypeStr=NOutDataTypeStr
  Integral Gain : Gain  DisableCoverage=on  Gain=I  ParamMin=IParamMin  ParamMax=IParamMax  ParamDataTypeStr=IParamDataTypeStr  OutMin=IOutMin  OutMax=IOutMax  OutDataTypeStr=IOutDataTypeStr
  Integrator : Integrator  ExternalReset=rising  InitialCondition=InitialConditionForIntegrator
  Product : Product
  Product1 : Product
  Product2 : Product
  Proportional Gain : Gain  Gain=P  ParamMin=PParamMin  ParamMax=PParamMax  ParamDataTypeStr=PParamDataTypeStr  OutMin=POutMin  OutMax=POutMax  OutDataTypeStr=POutDataTypeStr
  Saturation : Saturate  UpperLimit=UpperSaturationLimit  LowerLimit=LowerSaturationLimit  OutMin=SaturationOutMin  OutMax=SaturationOutMax  OutDataTypeStr=SaturationOutDataTypeStr
  Sum : Sum  Inputs=+++  AccumDataTypeStr=SumAccumDataTypeStr  OutMin=SumOutMin  OutMax=SumOutMax  OutDataTypeStr=SumOutDataTypeStr
  SumD : Sum  DisableCoverage=on  Inputs=|+-  AccumDataTypeStr=SumDAccumDataTypeStr  OutMin=SumDOutMin  OutMax=SumDOutMax  OutDataTypeStr=SumDOutDataTypeStr
  Switch : Switch  Criteria=u2 > Threshold  InputSameDT=on
  y : Outport  InitialOutput=0
  wires:
  p/1 -> Product/1
  u/1 -> Product2/2, Product1/2, Product/2
  Product1/1 -> Clamping circuit/2(preIntegrator), Switch/3
  Product2/1 -> SumD/1
  SumD/1 -> Filter Coefficient/1
  Filter Coefficient/1 -> Sum/3, Filter/1
  Filter/1 -> SumD/2
  Integrator/1 -> Sum/2
  Product/1 -> Sum/1
  RESET/1 -> Integrator/2, Filter/2
  Saturation/1 -> y/1
  Sum/1 -> Clamping circuit/1(preSat), Saturation/1
  Constant/1 -> Switch/1
  Clamping circuit/1(Clamp) -> Switch/2
  Switch/1 -> Integrator/1
  i/1 -> Product1/1
  d/1 -> Product2/1

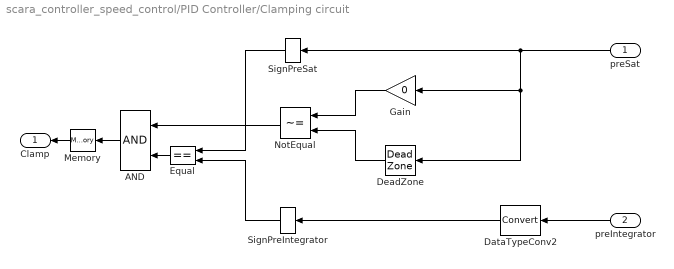
== system scara_controller_speed_control/PID Controller/Clamping circuit ==
  preSat : Inport
  preIntegrator : Inport  Port=2
  AND : Logic  DisableCoverage=on  OutDataTypeStr=boolean
  DataTypeConv2 : DataTypeConversion  DisableCoverage=on
  DeadZone : DeadZone  DisableCoverage=on  LowerValue=LowerSaturationLimit  UpperValue=UpperSaturationLimit
  Equal : RelationalOperator  DisableCoverage=on  Operator===  OutDataTypeStr=boolean
  Gain : Gain  DisableCoverage=on  Gain=0  SaturateOnIntegerOverflow=on  OutDataTypeStr=Inherit: Same as input  ParamDataTypeStr=Inherit: Same as input
  Memory : Memory  DisableCoverage=on
  NotEqual : RelationalOperator  DisableCoverage=on  Operator=~=  OutDataTypeStr=boolean
  SignPreIntegrator : Signum  DisableCoverage=on
  SignPreSat : Signum  DisableCoverage=on
  Clamp : Outport
  wires:
  preSat/1 -> DeadZone/1, Gain/1, SignPreSat/1
  preIntegrator/1 -> DataTypeConv2/1
  DataTypeConv2/1 -> SignPreIntegrator/1
  Gain/1 -> NotEqual/1
  DeadZone/1 -> NotEqual/2
  SignPreSat/1 -> Equal/1
  NotEqual/1 -> AND/1
  SignPreIntegrator/1 -> Equal/2
  Equal/1 -> AND/2
  AND/1 -> Memory/1
  Memory/1 -> Clamp/1
